simulink model "test"  (R2024b)
settings: Solver=VariableStepAuto  StartTime=0.0  StopTime=100  RelTol=1e-3
undefined symbols (not defined in the file or in its folder): Ion, Lithium
libraries: spsDiodeLib x6, spsIdealSwitchLib x6, spsBatteryLib x4, spsSeriesRLCBranchLib x4, spsVoltageMeasurementLib x2, spsCurrentMeasurementLib x1, spsPWMGenerator2LevelLib x1, sps_lib x1
settings Model: Creator=yeswa  LastModifiedBy=yeswa

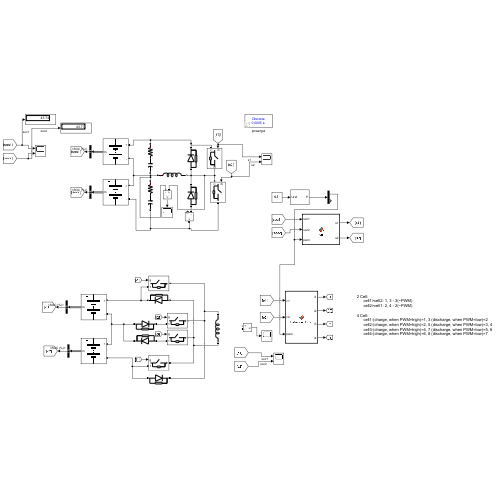
[thumbnail: Simulink's stored preview of the top-level diagram]
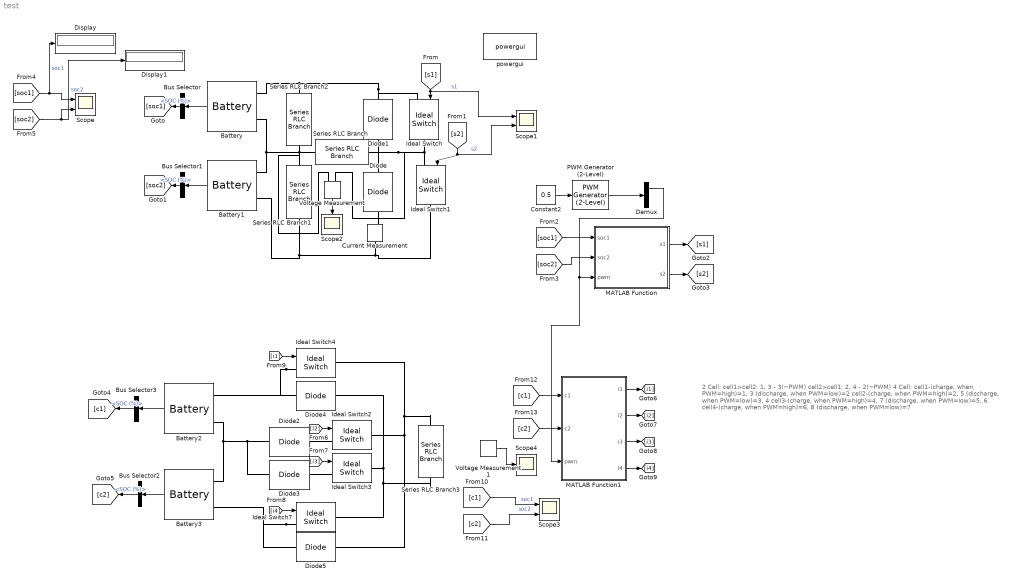
== system test ==
  note: 2 Cell:
      | cell1>cell2: 1, 3 - 3(~PWM)
      | cell2>cell1: 2, 4 - 2(~PWM)
      |
      | 4 Cell:
      | cell1-(charge, when PWM=high)=1, 3 (discharge, when PWM=low)=2
      | cell2-(charge, when PWM=high)=2, 5 (discharge, when PWM=low)=3, 4
      | cell3-(charge, when PWM=high)=4, 7 (discharge, when PWM=low)=5, 6
      | cell4-(charge, when PWM=high)=6, 8 (discharge, when PWM=low)=7
  Battery : spsBatteryLib/Battery  BatType=Lithium-Ion  NomV=3.7  NomQ=5.4  SOC=50  Batt_Tr=30  PresetModel=on  MaxQ=5.4  MinV=2.775  FullV=4.3068  Dis_rate=2.3478  R=0.0068519  Normal_OP=4.8835  expZone="[3.9974      0.2653]"
  Battery1 : spsBatteryLib/Battery  BatType=Lithium-Ion  NomV=3.7  NomQ=5.4  SOC=40  Batt_Tr=30  PresetModel=on  MaxQ=5.4  MinV=2.775  FullV=4.3068  Dis_rate=2.3478  R=0.0068519  Normal_OP=4.8835  expZone="[3.9974      0.2653]"
  Battery2 : spsBatteryLib/Battery  BatType=Lithium-Ion  NomV=3.7  NomQ=5.4  SOC=50  Batt_Tr=30  PresetModel=on  MaxQ=5.4  MinV=2.775  FullV=4.3068  Dis_rate=2.3478  R=0.0068519  Normal_OP=4.8835  expZone="[3.9974      0.2653]"
  Battery3 : spsBatteryLib/Battery  BatType=Lithium-Ion  NomV=3.7  NomQ=5.4  SOC=40  Batt_Tr=30  PresetModel=on  MaxQ=5.4  MinV=2.775  FullV=4.3068  Dis_rate=2.3478  R=0.0068519  Normal_OP=4.8835  expZone="[3.9974      0.2653]"
  Bus Selector{,1..3} (4 alike) : BusSelector  OutputSignals=SOC (%)
  Constant2 : Constant  Value=0.5
  Current Measurement : spsCurrentMeasurementLib/Current Measurement  PhasorSimulation=off  OutputType=Complex  PSBequivalent=0
  Demux : Demux  Outputs=2
  Diode{,1..5} (6 alike) : spsDiodeLib/Diode  Ron=0.001  Lon=0  Vf=0.8  IC=0  UseSnubber=0  Rs=500  Cs=250e-9  Measurements=off
  Display : Display
  Display1 : Display
  Ideal Switch{,1..4,7} (6 alike) : spsIdealSwitchLib/Ideal Switch  Ron=0.001  Lon=0  IC=0  Rs=1e5  Cs=inf  Measurements=off
  MATLAB Function : MATLAB Function  TreatAsAtomicUnit=on
  MATLAB Function1 : MATLAB Function  TreatAsAtomicUnit=on
  PWM Generator (2-Level) : spsPWMGenerator2LevelLib/PWM Generator (2-Level)  ModulatorType=Single-phase half-bridge (2 pulses)  ModulatorMode=Unsynchronized  Fc=25  Pc=0  nF=27  MinMax="[ -1  1 ]"  SamplingTechnique=Natural  ModulatingSignals=off  m=0.8  Freq=60  Phase=0  Ts=0  ShowCarrierOutport=off
  Scope : Scope  NumInputPorts=2
  Scope1 : Scope  NumInputPorts=2
  Scope2 : Scope
  Scope3 : Scope  NumInputPorts=2
  Scope4 : Scope
  Series RLC Branch : spsSeriesRLCBranchLib/Series RLC Branch  LConnTagsString=__new0  RConnTagsString=__new0  BranchType=L  Resistance=1  Inductance=1e-3  SetiL0=off  InitialCurrent=0  Capacitance=1e-6  Setx0=off  InitialVoltage=0  Measurements=None
  Series RLC Branch1 : spsSeriesRLCBranchLib/Series RLC Branch  LConnTagsString=__new0  RConnTagsString=__new0  BranchType=RC  Resistance=1  Inductance=1e-3  SetiL0=off  InitialCurrent=0  Capacitance=1e-6  Setx0=off  InitialVoltage=0  Measurements=None
  Series RLC Branch2 : spsSeriesRLCBranchLib/Series RLC Branch  LConnTagsString=__new0  RConnTagsString=__new0  BranchType=RC  Resistance=1  Inductance=1e-3  SetiL0=off  InitialCurrent=0  Capacitance=1e-6  Setx0=off  InitialVoltage=0  Measurements=None
  Series RLC Branch3 : spsSeriesRLCBranchLib/Series RLC Branch  LConnTagsString=__new0  RConnTagsString=__new0  BranchType=L  Resistance=1  Inductance=1e-3  SetiL0=off  InitialCurrent=0  Capacitance=1e-6  Setx0=off  InitialVoltage=0  Measurements=None
  Voltage Measurement : spsVoltageMeasurementLib/Voltage Measurement  PhasorSimulation=off  OutputType=Complex  PSBequivalent=0
  Voltage Measurement1 : spsVoltageMeasurementLib/Voltage Measurement  PhasorSimulation=off  OutputType=Complex  PSBequivalent=0
  powergui : sps_lib/powergui  Priority=1  SimulationMode=Discrete  SampleTime=50e-5  frequency=60  Iterations=50  frequencyindice=0  Pbase=100e6  ErrMax=1e-4  UnitsV=kV  UnitsW=MW  buscounter=0  FunctionMessages=off  echomessages=off  EnableUseOfTLC=off  CurrentSourceSwitches=off  DisableSnubberDevices=off  DisableRonSwitches=off  DisableVfSwitches=off  DisplayEquations=off  AutomaticDiscreteSolvers=off  SolverType=Tustin/Backward Euler (TBE)  Interpol=off  ExternalGateDelay=off  methode=off  Ts=100  x0status=blocks  SPID=on  SwTol=0  HookPort=off  NonlinearTolerance=1e-4  nMaxIteration=100  ContinueOnMaxIteration=off  RestoreLinks=warning  ResistiveCurrentMeasurement=off  Frange=[0:2:500]  Ylog=off  Xlog=on  ShowGrid=off  save=off  variable=ZData  structure=0  ZoomFFT=off  StartTime=0.0  cycles=1  DisplayStyle=1  fundamental=60  FreqAxis=off  MaxFrequency=1000  frequencyindicesteady=1  RmsSteady=1  display=off
  wires:
  Battery/1 -> Bus Selector/1
  Bus Selector/1 -> [soc1]  "<SOC (%)>"
  Bus Selector1/1 -> [soc2]  "<SOC (%)>"
  Battery1/1 -> Bus Selector1/1
  [s1] -> Scope1/1, Ideal Switch/1  "s1"
  [s2] -> Scope1/2, Ideal Switch1/1  "s2"
  Demux/1 -> MATLAB Function1/3(pwm), MATLAB Function/3(pwm)
  PWM Generator (2-Level)/1 -> Demux/1
  MATLAB Function/2(s2) -> [s2]
  [soc1] -> MATLAB Function/1(soc1)
  [soc2] -> MATLAB Function/2(soc2)
  MATLAB Function/1(s1) -> [s1]
  Constant2/1 -> PWM Generator (2-Level)/1
  [soc1] -> Display/1, Scope/1  "soc1"
  [soc2] -> Display1/1, Scope/2  "soc2"
  Voltage Measurement/1 -> Scope2/1
  [i2] -> Ideal Switch2/1
  [i3] -> Ideal Switch3/1
  [i1] -> Ideal Switch4/1
  [i4] -> Ideal Switch7/1
  Bus Selector3/1 -> [c1]  "<SOC (%)>"
  Bus Selector2/1 -> [c2]  "<SOC (%)>"
  Battery2/1 -> Bus Selector3/1
  Battery3/1 -> Bus Selector2/1
  [c1] -> Scope3/1  "soc1"
  [c2] -> Scope3/2  "soc2"
  [c1] -> MATLAB Function1/1(c1)
  [c2] -> MATLAB Function1/2(c2)
  MATLAB Function1/1(i1) -> [i1]
  MATLAB Function1/2(i2) -> [i2]
  MATLAB Function1/4(i4) -> [i4]
  MATLAB Function1/3(i3) -> [i3]
  Voltage Measurement1/1 -> Scope4/1
  connections:
  Battery1/LConn1 -- Voltage Measurement/LConn2 -- Series RLC Branch1/LConn1 -- Series RLC Branch2/RConn1 -- Series RLC Branch/LConn1 -- Battery/LConn2
  Battery/LConn1 -- Series RLC Branch2/LConn1 -- Ideal Switch/LConn1 -- Diode1/RConn1
  Battery1/LConn2 -- Series RLC Branch1/RConn1 -- Current Measurement/LConn1 -- Ideal Switch1/RConn1
  Ideal Switch/RConn1 -- Diode1/LConn1 -- Series RLC Branch/RConn1 -- Diode/RConn1 -- Voltage Measurement/LConn1 -- Ideal Switch1/LConn1
  Current Measurement/RConn1 -- Diode/LConn1
  Diode2/LConn1 -- Battery2/LConn2 -- Battery3/LConn1 -- Diode3/RConn1
  Ideal Switch2/LConn1 -- Diode2/RConn1
  Diode3/LConn1 -- Ideal Switch3/LConn1
  Ideal Switch4/LConn1 -- Battery2/LConn1 -- Diode4/RConn1
  Ideal Switch7/LConn1 -- Diode5/LConn1 -- Battery3/LConn2
  Ideal Switch7/RConn1 -- Series RLC Branch3/RConn1 -- Ideal Switch3/RConn1 -- Diode4/LConn1
  Diode5/RConn1 -- Ideal Switch2/RConn1 -- Series RLC Branch3/LConn1 -- Ideal Switch4/RConn1

== matlab function test/MATLAB Function1 ==
  settings: updateMethod=DISCRETE
  data: c1 input; i1 output; c2 input; pwm input; i2 output; i3 output; i4 output
function [i1, i2, i3, i4] = balance_logic(c1, c2, pwm)
% Inputs:
%   c1   -> SOC of cell1 (%)
%   c2   -> SOC of cell2 (%)
%   pwm  -> PWM input (0 or 1), 500 Hz, 1-phase half-bridge
%
% Outputs:
%   i1,i2,i3,i4 -> control signals for switches

% Persistent step counter
persistent stepCount
if isempty(stepCount)
    stepCount = int32(0);
end

% Initialize outputs
i1 = 0; i2 = 0; i3 = 0; i4 = 0;

% Threshold to avoid chatter
threshold = 0.5; % SOC % difference

% Balancing logic
if c1 > c2 + threshold
    % Cell1 has higher SOC
    if pwm == 1
        i1 = 1; 
        i3 = 1;
    else
        i3 = 1;
    end

elseif c2 > c1 + threshold
    % Cell2 has higher SOC
    if pwm == 1
        i2 = 1; 
        i4 = 1;
    else
        i2 = 1;
    end

else
    % Balanced
    i1 = 0; i2 = 0; i3 = 0; i4 = 0;
end

% Increment step counter
stepCount = stepCount + 1;

% Debug messages (for first 500 steps only)
if stepCount <= 500
    fprintf('Step %d | SOC1=%.2f | SOC2=%.2f | PWM=%d | i1=%d i2=%d i3=%d i4=%d\n', ...
        int32(stepCount), c1, c2, int32(pwm), int32(i1), int32(i2), int32(i3), int32(i4));
end

end

== matlab function test/MATLAB Function ==
  data: soc1 input; s1 output; soc2 input; s2 output; pwm input
function [s1, s2] = fcn(soc1, soc2, pwm)

if soc2<soc1
    s1=pwm;
    s2=0;
elseif soc1<soc2
    s1=0;
    s2=pwm;
else
    s1=0;
    s2=0;
end
